simulink model "lyapunovControl"  (R2015a)
settings: Solver=ode3  StartTime=0.0  StopTime=50  FixedStep=0.01  RelTol=1e-3
undefined symbols (not defined in the file or in its folder): lyapu
libraries: simulink x2
settings Model: CovModelRefEnable=off  Creator=Subodh  LastModifiedBy=smishra
settings DataIOCC: SaveFormat=Dataset
settings HardwareCC: ProdBitPerPointer=64  ProdLargestAtomicFloat=Float  ProdIntDivRoundTo=Zero  ProdEndianess=LittleEndian  ProdHWDeviceType=Specified
settings GRTTargetCC: GeneratePreprocessorConditionals=Use local settings

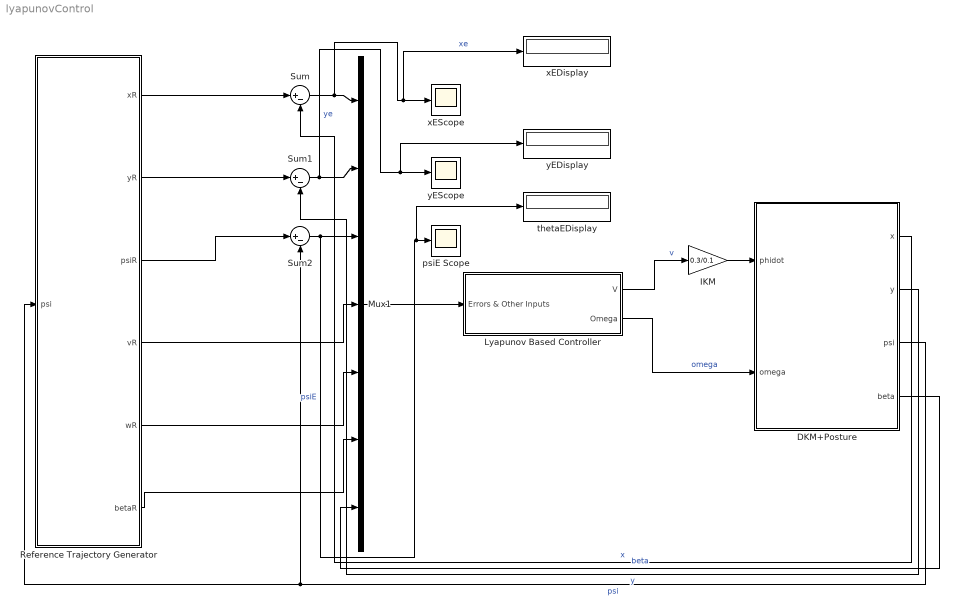
== system lyapunovControl ==
  DKM+Posture : Subsystem
  IKM : Gain  Gain=0.3/0.1
  Lyapunov Based Controller : Subsystem
  Mux1 : Mux  Inputs=7
  Reference Trajectory Generator : Subsystem
  Sum : Sum  Inputs=|+-
  Sum1 : Sum  Inputs=|+-
  Sum2 : Sum  Inputs=|+-
  psiE Scope : Scope
      settings: YMin=-0.00028  YMax=0.00003  SaveName=ScopeData2
  thetaEDisplay : Display
  xEDisplay : Display
  xEScope : Scope
      settings: YMin=-0.51889  YMax=0.6854
  yEDisplay : Display
  yEScope : Scope
      settings: YMin=-1.94871  YMax=0.53837
  wires:
  Reference Trajectory Generator/4(vR) -> Mux1/4
  Reference Trajectory Generator/5(wR) -> Mux1/5
  Reference Trajectory Generator/6(betaR) -> Mux1/6
  Reference Trajectory Generator/1(xR) -> Sum/1
  Sum/1 -> xEDisplay/1, xEScope/1, Mux1/1  "xe"
  Reference Trajectory Generator/2(yR) -> Sum1/1
  Sum1/1 -> yEDisplay/1, yEScope/1, Mux1/2  "ye"
  Reference Trajectory Generator/3(psiR) -> Sum2/1
  Sum2/1 -> thetaEDisplay/1, psiE Scope/1, Mux1/3  "psiE"
  DKM+Posture/1(x) -> Sum/2  "x"
  DKM+Posture/2(y) -> Sum1/2  "y"
  DKM+Posture/3(psi) -> Reference Trajectory Generator/1(psi), Sum2/2  "psi"
  DKM+Posture/4(beta) -> Mux1/7  "beta"
  Mux1/1 -> Lyapunov Based Controller/1(Errors & Other Inputs)
  Lyapunov Based Controller/2(Omega) -> DKM+Posture/2(omega)  "omega"
  IKM/1 -> DKM+Posture/1(phidot)
  Lyapunov Based Controller/1(V) -> IKM/1  "v"

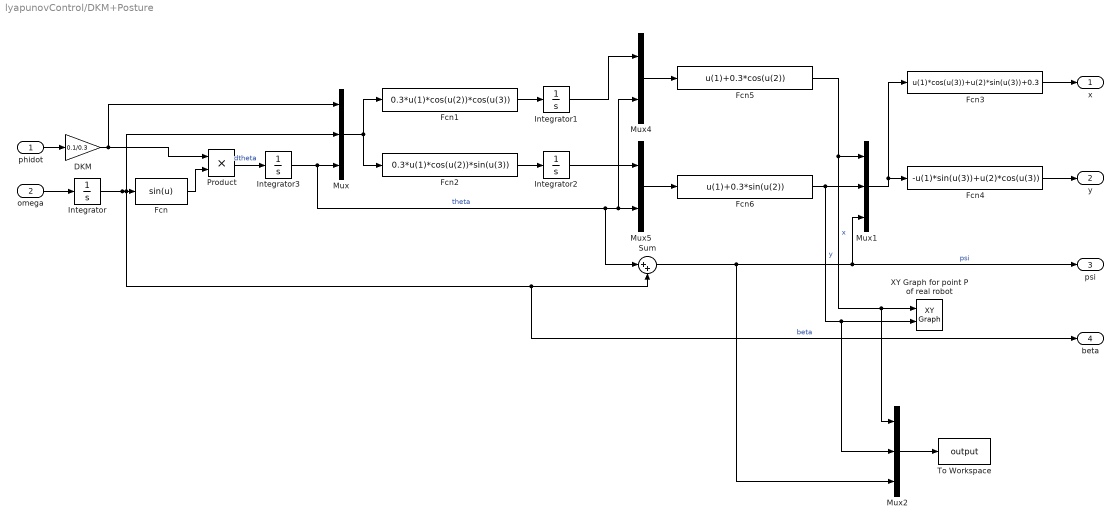
== system lyapunovControl/DKM+Posture ==
  phidot : Inport
  omega : Inport  Port=2
  DKM : Gain  Gain=0.1/0.3
  Fcn : Fcn  Expr=sin(u)
  Fcn1 : Fcn  Expr=0.3*u(1)*cos(u(2))*cos(u(3))
  Fcn2 : Fcn  Expr=0.3*u(1)*cos(u(2))*sin(u(3))
  Fcn3 : Fcn  Expr=u(1)*cos(u(3))+u(2)*sin(u(3))+0.3
  Fcn4 : Fcn  Expr=-u(1)*sin(u(3))+u(2)*cos(u(3))
  Fcn5 : Fcn  Expr=u(1)+0.3*cos(u(2))
  Fcn6 : Fcn  Expr=u(1)+0.3*sin(u(2))
  Integrator : Integrator
  Integrator1 : Integrator  InitialCondition=2.3
  Integrator2 : Integrator
  Integrator3 : Integrator  InitialCondition=pi
  Mux : Mux  Inputs=3
  Mux1 : Mux  Inputs=3
  Mux2 : Mux  Inputs=3
  Mux4 : Mux  Inputs=2
  Mux5 : Mux  Inputs=2
  Product : Product
  Sum : Sum  Inputs=|++
  To Workspace : ToWorkspace  VariableName=output  SampleTime=-1
  XY Graph for point P of real robot : simulink/Sinks/XY Graph  xmin=-2  xmax=2  ymin=-2  ymax=2  st=-1
  x : Outport
  y : Outport  Port=2
  psi : Outport  Port=3
  beta : Outport  Port=4
  wires:
  Mux5/1 -> Fcn6/1
  Integrator1/1 -> Mux4/1
  Mux4/1 -> Fcn5/1
  Integrator2/1 -> Mux5/1
  Fcn/1 -> Product/2
  omega/1 -> Integrator/1
  Fcn2/1 -> Integrator2/1
  Fcn1/1 -> Integrator1/1
  Integrator3/1 -> Sum/1, Mux4/2, Mux5/2, Mux/3  "theta"
  Product/1 -> Integrator3/1  "dtheta"
  Integrator/1 -> Mux/2, beta/1, Sum/2, Fcn/1  "beta"
  Mux/1 -> Fcn2/1, Fcn1/1
  Sum/1 -> Mux2/3, Mux1/3, psi/1  "psi"
  Fcn5/1 -> Mux2/1, XY Graph for point P of real robot/1, Mux1/1  "x"
  Fcn6/1 -> Mux2/2, XY Graph for point P of real robot/2, Mux1/2  "y"
  Fcn3/1 -> x/1
  Mux1/1 -> Fcn4/1, Fcn3/1
  Fcn4/1 -> y/1
  Mux2/1 -> To Workspace/1
  phidot/1 -> DKM/1
  DKM/1 -> Mux/1, Product/1

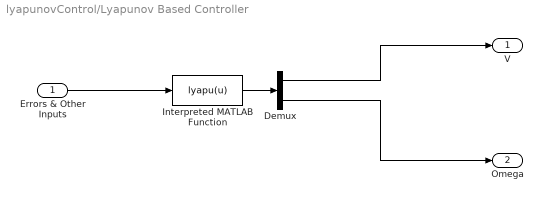
== system lyapunovControl/Lyapunov Based Controller ==
  Errors & Other Inputs : Inport
  Demux : Demux  Outputs=2
  Interpreted MATLAB Function : MATLABFcn  MATLABFcn=lyapu(u)
  V : Outport
  Omega : Outport  Port=2
  wires:
  Errors & Other Inputs/1 -> Interpreted MATLAB Function/1
  Demux/2 -> Omega/1
  Demux/1 -> V/1
  Interpreted MATLAB Function/1 -> Demux/1

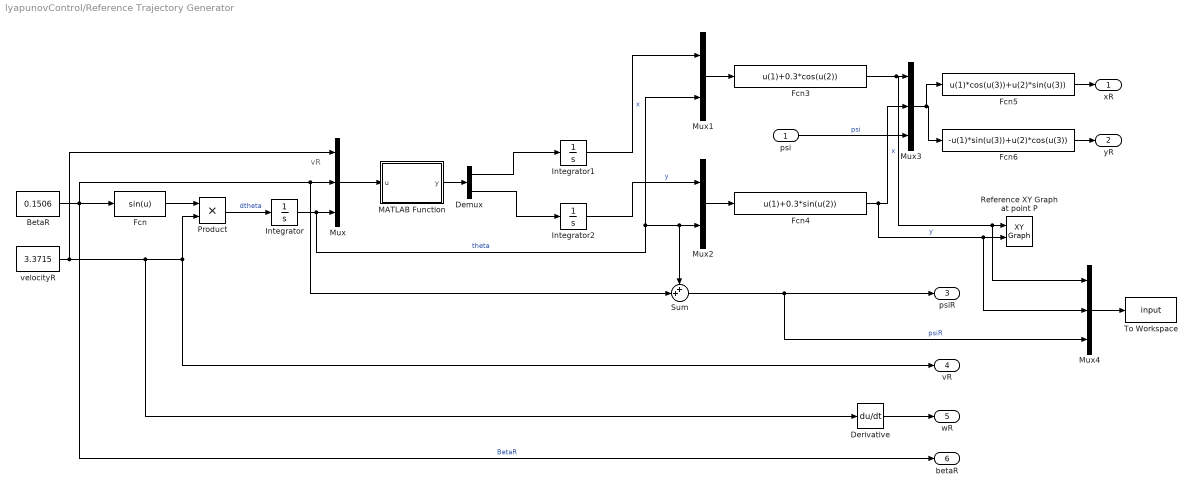
== system lyapunovControl/Reference Trajectory Generator ==
  note: vR
  psi : Inport
  BetaR : Constant  Value=0.1506
  Demux : Demux  Outputs=2
  Derivative : Derivative
  Fcn : Fcn  Expr=sin(u)
  Fcn3 : Fcn  Expr=u(1)+0.3*cos(u(2))
  Fcn4 : Fcn  Expr=u(1)+0.3*sin(u(2))
  Fcn5 : Fcn  Expr=u(1)*cos(u(3))+u(2)*sin(u(3))
  Fcn6 : Fcn  Expr=-u(1)*sin(u(3))+u(2)*cos(u(3))
  Integrator : Integrator  InitialCondition=pi/2
  Integrator1 : Integrator  InitialCondition=sqrt(4-0.09)
  Integrator2 : Integrator
  MATLAB Function : MATLAB Function  TreatAsAtomicUnit=on
  Mux : Mux  Inputs=3
  Mux1 : Mux  Inputs=2
  Mux2 : Mux  Inputs=2
  Mux3 : Mux  Inputs=3
  Mux4 : Mux  Inputs=3
  Product : Product
  Reference XY Graph at point P : simulink/Sinks/XY Graph  xmin=-2  xmax=2  ymin=-2  ymax=2  st=-1
  Sum : Sum  Inputs=++|
  To Workspace : ToWorkspace  VariableName=input  SampleTime=-1
  velocityR : Constant  Value=3.3715
  xR : Outport
  yR : Outport  Port=2
  psiR : Outport  Port=3
  vR : Outport  Port=4
  wR : Outport  Port=5
  betaR : Outport  Port=6
  wires:
  Mux2/1 -> Fcn4/1
  Product/1 -> Integrator/1  "dtheta"
  Fcn/1 -> Product/1
  BetaR/1 -> betaR/1, Mux/2, Sum/2, Fcn/1  "BetaR"
  velocityR/1 -> Derivative/1, vR/1, Product/2, Mux/1
  Demux/1 -> Integrator1/1
  Demux/2 -> Integrator2/1
  Integrator1/1 -> Mux1/1  "x"
  Mux1/1 -> Fcn3/1
  Integrator/1 -> Mux1/2, Sum/1, Mux2/2, Mux/3  "theta"
  Integrator2/1 -> Mux2/1  "y"
  Sum/1 -> Mux4/3, psiR/1  "psiR"
  Derivative/1 -> wR/1
  Fcn3/1 -> Mux4/1, Reference XY Graph at point P/1, Mux3/1  "x"
  Fcn4/1 -> Mux4/2, Reference XY Graph at point P/2, Mux3/2  "y"
  psi/1 -> Mux3/3  "psi"
  Mux3/1 -> Fcn5/1, Fcn6/1
  Fcn5/1 -> xR/1
  Fcn6/1 -> yR/1
  Mux4/1 -> To Workspace/1
  Mux/1 -> MATLAB Function/1(u)
  MATLAB Function/1(y) -> Demux/1

== matlab function lyapunovControl/Reference Trajectory Generator/MATLAB Function ==
  data: u input; y output
function y = fcn(u)
%#codegen
a=0.3;
y=zeros(2,1);
y(1)=a*u(1)*cos(u(2))*cos(u(3));
y(2)=a*u(1)*cos(u(2))*sin(u(3));
y=y(:);
